simulink model "sys_ctrl_obs"  (Simulink 7.6)
settings: Solver=ode45  StartTime=0.0  StopTime=10.0  MaxStep=0.01  RelTol=1e-3
values from neighbouring files (symbols this model uses):
  A = [0 1;-k/m -h/m]    [ctrl2.m]    (also in ctrl_obs_BUONO.m = [2 3;4 1]; es1.m = [2 3;4 1])
  B = [0;1/m]    [ctrl2.m]    (also in ctrl_obs_BUONO.m = [1;0]; es1.m = [1;0])
  C = [1 0]    [ctrl2.m]    (also in ctrl_obs_BUONO.m; es1.m)
  D = 0    [ctrl2.m]    (also in ctrl_obs_BUONO.m; es1.m)
  K = -place(A,B,aval_desiderati)    [ctrl2.m]    (also in ctrl_obs_BUONO.m = -place(A,B,aval_des); es1.m)
  L = -place(A',C',aval_obs_des)'    [ctrl_obs_BUONO.m]
  ueq = 3    [ctrl2.m]    (also in ctrl_obs_BUONO.m = 1; es1.m = 1)
  x0 = [1;0]    [ctrl2.m]    (also in ctrl_obs_BUONO.m = [1;1]; es1.m = [1;1])
  x0o = [0;0]    [ctrl_obs_BUONO.m]
  xeq = [0;0]    [ctrl2.m]    (also in ctrl_obs_BUONO.m; es1.m)
libraries: simulink x2
settings Model: Creator=professore  LastModifiedBy=patrizio

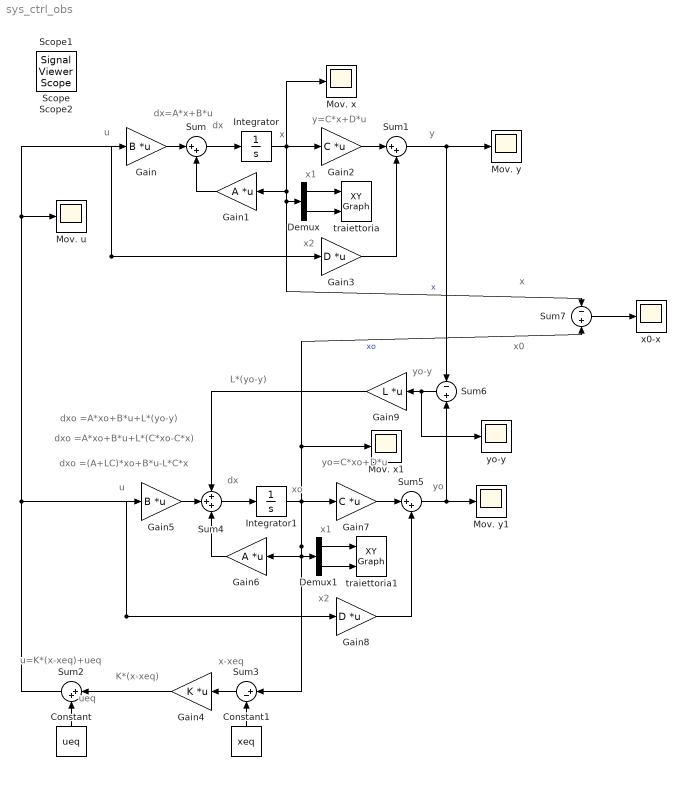
== system sys_ctrl_obs ==
  note: dx=A*x+B*u
  note: y=C*x+D*u
  note: u=K*(x-xeq)+ueq
  note: dx
  note: x
  note: u
  note: K*(x-xeq)
  note: ueq
  note: x-xeq
  note: x1
  note: x2
  note: dxo =A*xo+B*u+L*(yo-y)
  note: yo=C*xo+D*u
  note: dx
  note: xo
  note: u
  note: x1
  note: x2
  note: y
  note: yo
  note: yo-y
  note: L*(yo-y)
  note: dxo =A*xo+B*u+L*(C*xo-C*x)
  note: dxo =(A+LC)*xo+B*u-L*C*x
  note: x
  note: x0
  Constant : Constant  Value=ueq
  Constant1 : Constant  Value=xeq
  Demux : Demux  Outputs=2
  Demux1 : Demux  Outputs=2
  Gain : Gain  Gain=B  Multiplication=Matrix(K*u)
  Gain1 : Gain  Gain=A  Multiplication=Matrix(K*u)
  Gain2 : Gain  Gain=C  Multiplication=Matrix(K*u)
  Gain3 : Gain  Gain=D  Multiplication=Matrix(K*u)
  Gain4 : Gain  Gain=K  Multiplication=Matrix(K*u)
  Gain5 : Gain  Gain=B  Multiplication=Matrix(K*u)
  Gain6 : Gain  Gain=A  Multiplication=Matrix(K*u)
  Gain7 : Gain  Gain=C  Multiplication=Matrix(K*u)
  Gain8 : Gain  Gain=D  Multiplication=Matrix(K*u)
  Gain9 : Gain  Gain=L  Multiplication=Matrix(K*u)
  Integrator : Integrator  InitialCondition=x0
  Integrator1 : Integrator  InitialCondition=x0o
  Mov. u : Scope
      settings: SaveName=ScopeData2
  Mov. x : Scope
  Mov. x1 : Scope
      settings: SaveName=ScopeData3
  Mov. y : Scope
  Mov. y1 : Scope
      settings: SaveName=ScopeData4
  Sum{,1..2,5} (4 alike) : Sum  Inputs=|++
  Sum3 : Sum  Inputs=|+-
  Sum4 : Sum  Inputs=+++
  Sum6 : Sum  Inputs=-+
  Sum7 : Sum  Inputs=-+
  traiettoria : simulink/Sinks/XY Graph  SystemSampleTime=-1  xmin=1  xmax=1.5  ymin=0  ymax=2  st=-1
  traiettoria1 : simulink/Sinks/XY Graph  SystemSampleTime=-1  xmin=1  xmax=1.5  ymin=0  ymax=2  st=-1
  x0-x : Scope
      settings: SaveName=ScopeData6
  yo-y : Scope
      settings: SaveName=ScopeData5
  Scope : SignalViewerScope  IOType=viewer  ZoomMode=xonly  RefreshTime=0.035000
  Scope1 : SignalViewerScope  IOType=viewer  ZoomMode=xonly  RefreshTime=0.035000
  Scope2 : SignalViewerScope  IOType=viewer  RefreshTime=0.035000
      settings: SaveName=ScopeData2
  wires:
  Gain/1 -> Sum/1
  Gain1/1 -> Sum/2
  Sum/1 -> Integrator/1
  Integrator/1 -> Gain2/1, Gain1/1, Demux/1, Sum7/1, Mov. x/1  "x"
  Gain2/1 -> Sum1/1
  Gain3/1 -> Sum1/2
  Gain4/1 -> Sum2/1
  Constant/1 -> Sum2/2
  Sum3/1 -> Gain4/1
  Constant1/1 -> Sum3/2
  Sum2/1 -> Gain/1, Gain3/1, Mov. u/1, Gain5/1, Gain8/1
  Sum1/1 -> Mov. y/1, Sum6/1
  Demux/1 -> traiettoria/1
  Demux/2 -> traiettoria/2
  Sum4/1 -> Integrator1/1
  Integrator1/1 -> Gain7/1, Gain6/1, Demux1/1, Sum3/1, Mov. x1/1, Sum7/2  "xo"
  Gain7/1 -> Sum5/1
  Gain8/1 -> Sum5/2
  Sum5/1 -> Mov. y1/1, Sum6/2
  Demux1/1 -> traiettoria1/1
  Demux1/2 -> traiettoria1/2
  Sum6/1 -> Gain9/1, yo-y/1
  Gain9/1 -> Sum4/1
  Gain6/1 -> Sum4/3
  Gain5/1 -> Sum4/2
  Sum7/1 -> x0-x/1
